simulink model "PDregulatorQ"  (R2019b)
settings: Solver=FixedStepDiscrete  StartTime=0.0  StopTime=inf  FixedStep=0.01  RelTol=1e-3
values from neighbouring files (symbols this model uses):
  Kd = 0.1    [LetterN.mat]    (also in initNew.m; panda.m)
  Kp = 10    [LetterN.mat]    (also in initNew.m; panda.m)
libraries: simulink_extras x2, simulink x2, xpcutilitieslib x2, xpcrtudplib x2
settings Model: EnablePacing=on  Creator=Aljaz  LastModifiedBy=Aljaz

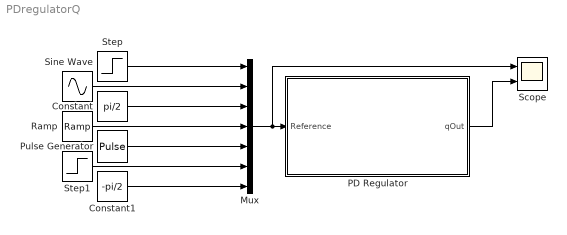
== system PDregulatorQ ==
  Constant : Constant  Value=pi/2
  Constant1 : Constant  Value=-pi/2
  Mux : Mux  Inputs=7
  PD Regulator : Subsystem
  Pulse Generator : DiscretePulseGenerator  PulseType=Time based  Amplitude=pi/3  Period=10  PulseWidth=20
  Ramp : simulink/Sources/Ramp  slope=-pi/1000  start=0  InitialOutput=0
  Scope : Scope  NumInputPorts=2
  Sine Wave : Sin  Amplitude=pi/3  Bias=pi/6  Frequency=0.5  SampleTime=0
  Step : Step  Time=5  Before=pi/2  After=pi/5  SampleTime=0
  Step1 : Step  Time=2  Before=pi/2  After=pi/4  SampleTime=0
  wires:
  Mux/1 -> Scope/1, PD Regulator/1(Reference)
  Step/1 -> Mux/1
  Sine Wave/1 -> Mux/2
  Constant/1 -> Mux/3
  Ramp/1 -> Mux/4
  Pulse Generator/1 -> Mux/5
  Step1/1 -> Mux/6
  Constant1/1 -> Mux/7
  PD Regulator/1(qOut) -> Scope/2

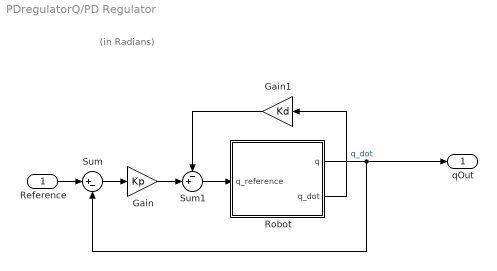
== system PDregulatorQ/PD Regulator ==
  note: (in Radians)
  Reference : Inport
  Gain : Gain  Gain=Kp
  Gain1 : Gain  Gain=Kd
  Robot : Subsystem
  Sum : Sum  Inputs=|+-
  Sum1 : Sum  Inputs=-+|
  qOut : Outport
  wires:
  Reference/1 -> Sum/1
  Sum1/1 -> Robot/1(q_reference)
  Gain/1 -> Sum1/2
  Sum/1 -> Gain/1
  Robot/1(q) -> qOut/1, Sum/2
  Gain1/1 -> Sum1/1
  Robot/2(q_dot) -> Gain1/1  "q_dot"

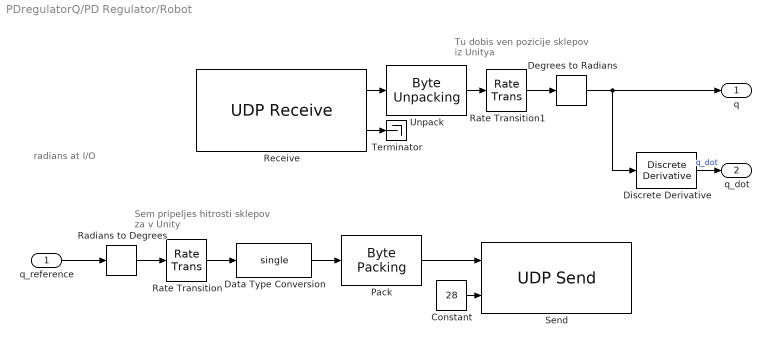
== system PDregulatorQ/PD Regulator/Robot ==
  note: radians at I/O
  note: Sem pripeljes hitrosti sklepov za v Unity
  note: Tu dobis ven pozicije sklepov iz Unitya
  q_reference : Inport
  Constant : Constant  Value=28
  Data Type Conversion : DataTypeConversion  OutDataTypeStr=single
  Degrees to Radians : simulink_extras/Transformations/Degrees to Radians
  Discrete Derivative : simulink/Discrete/Discrete Derivative  gainval=1  ICPrevScaledInput=0.0  OutMin=[]  OutMax=[]  OutDataType=fixdt(1, 16)  OutScaling=2^-10  DoSatur=off
  Pack : xpcutilitieslib/Byte Packing   MaskPackedDataType=uint8  MaskUnpackedDataTypes={'single'}  MaskAlignment=1
  Radians to Degrees : simulink_extras/Transformations/Radians to Degrees
  Rate Transition : RateTransition  InitialCondition=[0 0 0 0 0 0 0]
  Rate Transition1 : RateTransition
  Receive : xpcrtudplib/UDP Receive  ipAddressVal=Use host-target connection  localPort=25106  rcvWidth=7*4  rcvFmAny=off  fmAddress=127.0.0.1  rcvMulticast=off  multicastAddress={}  maxUDPQueue=8  sampleTime=0.01
      settings: SourceProductName=Simulink Real-Time
  Send : xpcrtudplib/UDP Send  ipAddressVal=Use host-target connection  localPort=-1  toAddress=127.0.0.1  toPort=25008  sampleTime=0.01
      settings: SourceProductName=Simulink Real-Time  SourceProductBaseCode=XP
  Terminator : Terminator
  Unpack : xpcutilitieslib/Byte Unpacking   MaskUnpackedDataTypes={'single'}  MaskUnpackedDataSizes={[7]}  MaskAlignment=1
      settings: SourceProductName=Simulink Real-Time  SourceProductBaseCode=XP
  q : Outport
  q_dot : Outport  Port=2
  wires:
  Constant/1 -> Send/2
  Pack/1 -> Send/1
  Receive/1 -> Unpack/1
  Rate Transition/1 -> Data Type Conversion/1
  Unpack/1 -> Rate Transition1/1
  Receive/2 -> Terminator/1
  Data Type Conversion/1 -> Pack/1
  Discrete Derivative/1 -> q_dot/1  "q_dot"
  Degrees to Radians/1 -> q/1, Discrete Derivative/1
  Rate Transition1/1 -> Degrees to Radians/1
  q_reference/1 -> Radians to Degrees/1
  Radians to Degrees/1 -> Rate Transition/1
